simulink model "ZN_P1P2P3"  (R2019b)
settings: Solver=VariableStepAuto  StartTime=0.0  StopTime=300  RelTol=1e-3
libraries: simulink x3
settings Model: Creator=dibakarrajbongshi  LastModifiedBy=HP

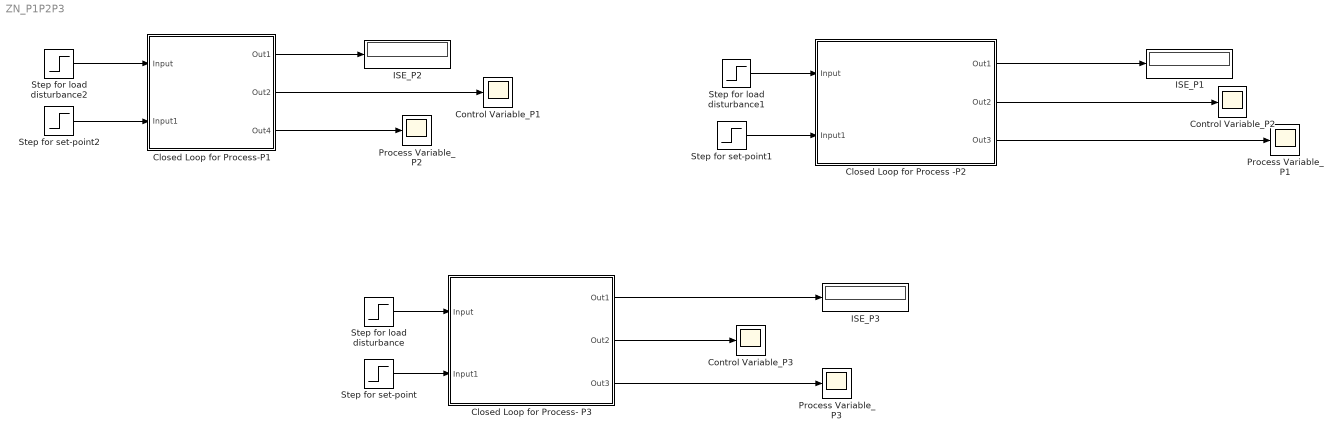
== system ZN_P1P2P3 ==
  Closed Loop for Process -P2 : Subsystem
  Closed Loop for Process- P3 : Subsystem
  Closed Loop for Process-P1 : Subsystem
  Control Variable_P1 : Scope
  Control Variable_P2 : Scope
  Control Variable_P3 : Scope
  ISE_P1 : Display
  ISE_P2 : Display
  ISE_P3 : Display
  Process Variable_P1 : Scope
  Process Variable_P2 : Scope
  Process Variable_P3 : Scope
  Step for load disturbance : Step  Time=0  After=0  SampleTime=0
  Step for load disturbance1 : Step  Time=0  After=0  SampleTime=0
  Step for load disturbance2 : Step  Time=0  After=0  SampleTime=0
  Step for set-point : Step  Time=0  SampleTime=0
  Step for set-point1 : Step  Time=0  SampleTime=0
  Step for set-point2 : Step  Time=0  SampleTime=0
  wires:
  Step for set-point2/1 -> Closed Loop for Process-P1/2(Input1)
  Closed Loop for Process-P1/3(Out4) -> Process Variable_P2/1
  Step for load disturbance2/1 -> Closed Loop for Process-P1/1(Input)
  Closed Loop for Process-P1/2(Out2) -> Control Variable_P1/1
  Closed Loop for Process-P1/1(Out1) -> ISE_P2/1
  Closed Loop for Process -P2/2(Out2) -> Control Variable_P2/1
  Step for load disturbance1/1 -> Closed Loop for Process -P2/1(Input)
  Closed Loop for Process -P2/3(Out3) -> Process Variable_P1/1
  Step for set-point1/1 -> Closed Loop for Process -P2/2(Input1)
  Closed Loop for Process -P2/1(Out1) -> ISE_P1/1
  Closed Loop for Process- P3/2(Out2) -> Control Variable_P3/1
  Closed Loop for Process- P3/3(Out3) -> Process Variable_P3/1
  Closed Loop for Process- P3/1(Out1) -> ISE_P3/1
  Step for load disturbance/1 -> Closed Loop for Process- P3/1(Input)
  Step for set-point/1 -> Closed Loop for Process- P3/2(Input1)

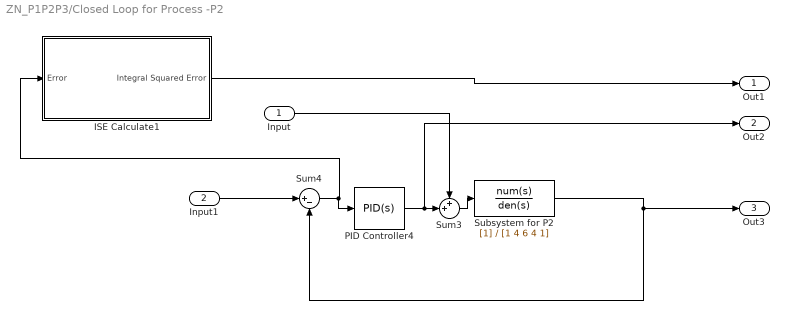
== system ZN_P1P2P3/Closed Loop for Process -P2 ==
  Input : Inport
  Input1 : Inport  Port=2
  ISE Calculate1 : Subsystem
  PID Controller4 : simulink/Continuous/PID Controller  Controller=PID  Form=Parallel  TimeDomain=Continuous-time  SampleTime=-1  IntegratorMethod=Forward Euler  FilterMethod=Forward Euler  ControllerParametersSource=internal  P=2.353  I=0.75  D=1.847  UseFilter=on  N=12.74  TunerSelectOption=Transfer Function Based (PID Tuner App)  InitialConditionSource=internal  InitialConditionForIntegrator=0  InitialConditionForFilter=0  DifferentiatorICPrevScaledInput=0  ExternalReset=none  TrackingMode=off  Kt=1  LimitOutput=off  UpperSaturationLimit=0.9  LowerSaturationLimit=0.1  LinearizeAsGain=on  AntiWindupMode=none  Kb=1  POutMin=[]  POutMax=[]  IOutMin=[]  IOutMax=[]  DOutMin=[]  DOutMax=[]  NOutMin=[]  NOutMax=[]  SumOutMin=[]  SumOutMax=[]  SaturationOutMin=[]  SaturationOutMax=[]  PParamMin=[]  PParamMax=[]  IParamMin=[]  IParamMax=[]  DParamMin=[]  DParamMax=[]  NParamMin=[]  NParamMax=[]  KbParamMin=[]  KbParamMax=[]  KtParamMin=[]  KtParamMax=[]  KbOutMin=[]  KbOutMax=[]  KtOutMin=[]  KtOutMax=[]  IntegratorOutMin=[]  IntegratorOutMax=[]  FilterOutMin=[]  FilterOutMax=[]  SumI1OutMin=[]  SumI1OutMax=[]  SumI2OutMin=[]  SumI2OutMax=[]  SumI3OutMin=[]  SumI3OutMax=[]  SumI4OutMin=[]  SumI4OutMax=[]  SumDOutMin=[]  SumDOutMax=[]  DifferentiatorOutMin=[]  DifferentiatorOutMax=[]  FilterDiffOutCoefMin=[]  FilterDiffOutCoefMax=[]  ReciprocalOutMin=[]  ReciprocalOutMax=[]  SumDenOutMin=[]  SumDenOutMax=[]  SumNumOutMin=[]  SumNumOutMax=[]  DivideOutMin=[]  DivideOutMax=[]  IntegratorContinuousStateAttributes=''  IntegratorStateMustResolveToSignalObject=off  IntegratorRTWStateStorageClass=Auto  FilterContinuousStateAttributes=''  FilterStateMustResolveToSignalObject=off  FilterRTWStateStorageClass=Auto  ParallelPVariant=InternalParameters  IdealPVariant=Disabled  IVariant=InternalParameters  DVariant=InternalParameters  IntegratorVariant=Continuous  SatVariant=Disabled  AWVariant=Passthrough  PCopyVariant=Disabled  TRVariant=Disabled  FdbkBlocksVariant=Forward  IdealPFdbkVariant=Disabled  SatFdbkVariant=Disabled  DerivativeFilterVariant=ContFilter  NVariant=InternalParameters  NCopyVariant=Disabled  FilterICVariant=InternalICsFilter  IntegratorICVariant=InternalICs  ExternalResetVariant=Disabled  TRSumVariant=Passthrough  SumFdbkVariant=Disabled  SumVariant=Sum_PID
  Subsystem for P2 : TransferFcn  Denominator=[1 4 6 4 1]
  Sum3 : Sum  Inputs=++|
  Sum4 : Sum  Inputs=|+-
  Out1 : Outport
  Out2 : Outport  Port=2
  Out3 : Outport  Port=3
  wires:
  PID Controller4/1 -> Out2/1, Sum3/2
  Input/1 -> Sum3/1
  Subsystem for P2/1 -> Out3/1, Sum4/2
  Sum4/1 -> PID Controller4/1, ISE Calculate1/1(Error)
  ISE Calculate1/1(Integral Squared Error) -> Out1/1
  Input1/1 -> Sum4/1
  Sum3/1 -> Subsystem for P2/1

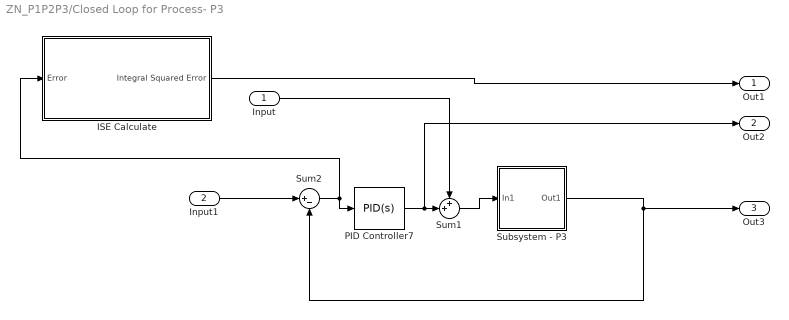
== system ZN_P1P2P3/Closed Loop for Process- P3 ==
  Input : Inport
  Input1 : Inport  Port=2
  ISE Calculate : Subsystem
  PID Controller7 : simulink/Continuous/PID Controller  Controller=PID  Form=Parallel  TimeDomain=Continuous-time  SampleTime=-1  IntegratorMethod=Forward Euler  FilterMethod=Forward Euler  ControllerParametersSource=internal  P=0.75  I=0.0382  D=3.6825  UseFilter=on  N=2.03666  TunerSelectOption=Transfer Function Based (PID Tuner App)  InitialConditionSource=internal  InitialConditionForIntegrator=0  InitialConditionForFilter=0  DifferentiatorICPrevScaledInput=0  ExternalReset=none  TrackingMode=off  Kt=1  LimitOutput=off  UpperSaturationLimit=0.9  LowerSaturationLimit=0.1  LinearizeAsGain=on  AntiWindupMode=none  Kb=1  POutMin=[]  POutMax=[]  IOutMin=[]  IOutMax=[]  DOutMin=[]  DOutMax=[]  NOutMin=[]  NOutMax=[]  SumOutMin=[]  SumOutMax=[]  SaturationOutMin=[]  SaturationOutMax=[]  PParamMin=[]  PParamMax=[]  IParamMin=[]  IParamMax=[]  DParamMin=[]  DParamMax=[]  NParamMin=[]  NParamMax=[]  KbParamMin=[]  KbParamMax=[]  KtParamMin=[]  KtParamMax=[]  KbOutMin=[]  KbOutMax=[]  KtOutMin=[]  KtOutMax=[]  IntegratorOutMin=[]  IntegratorOutMax=[]  FilterOutMin=[]  FilterOutMax=[]  SumI1OutMin=[]  SumI1OutMax=[]  SumI2OutMin=[]  SumI2OutMax=[]  SumI3OutMin=[]  SumI3OutMax=[]  SumI4OutMin=[]  SumI4OutMax=[]  SumDOutMin=[]  SumDOutMax=[]  DifferentiatorOutMin=[]  DifferentiatorOutMax=[]  FilterDiffOutCoefMin=[]  FilterDiffOutCoefMax=[]  ReciprocalOutMin=[]  ReciprocalOutMax=[]  SumDenOutMin=[]  SumDenOutMax=[]  SumNumOutMin=[]  SumNumOutMax=[]  DivideOutMin=[]  DivideOutMax=[]  IntegratorContinuousStateAttributes=''  IntegratorStateMustResolveToSignalObject=off  IntegratorRTWStateStorageClass=Auto  FilterContinuousStateAttributes=''  FilterStateMustResolveToSignalObject=off  FilterRTWStateStorageClass=Auto  ParallelPVariant=InternalParameters  IdealPVariant=Disabled  IVariant=InternalParameters  DVariant=InternalParameters  IntegratorVariant=Continuous  SatVariant=Disabled  AWVariant=Passthrough  PCopyVariant=Disabled  TRVariant=Disabled  FdbkBlocksVariant=Forward  IdealPFdbkVariant=Disabled  SatFdbkVariant=Disabled  DerivativeFilterVariant=ContFilter  NVariant=InternalParameters  NCopyVariant=Disabled  FilterICVariant=InternalICsFilter  IntegratorICVariant=InternalICs  ExternalResetVariant=Disabled  TRSumVariant=Passthrough  SumFdbkVariant=Disabled  SumVariant=Sum_PID
  Subsystem - P3 : Subsystem
  Sum1 : Sum  Inputs=++|
  Sum2 : Sum  Inputs=|+-
  Out1 : Outport
  Out2 : Outport  Port=2
  Out3 : Outport  Port=3
  wires:
  PID Controller7/1 -> Out2/1, Sum1/2
  Subsystem - P3/1(Out1) -> Out3/1, Sum2/2
  Sum2/1 -> PID Controller7/1, ISE Calculate/1(Error)
  ISE Calculate/1(Integral Squared Error) -> Out1/1
  Input1/1 -> Sum2/1
  Sum1/1 -> Subsystem - P3/1(In1)
  Input/1 -> Sum1/1

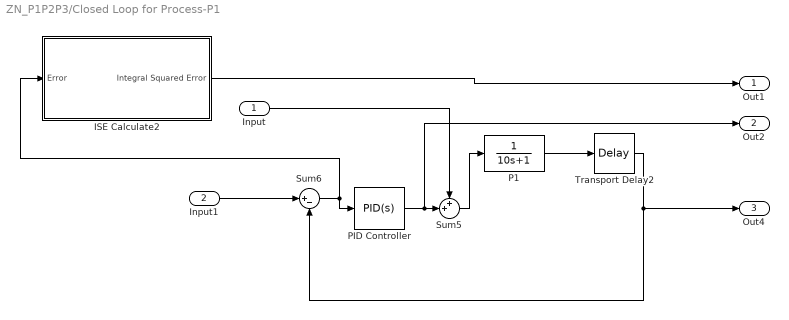
== system ZN_P1P2P3/Closed Loop for Process-P1 ==
  Input : Inport
  Input1 : Inport  Port=2
  ISE Calculate2 : Subsystem
  P1 : TransferFcn  Denominator=[10 1]
  PID Controller : simulink/Continuous/PID Controller  Controller=PID  Form=Parallel  TimeDomain=Continuous-time  SampleTime=-1  IntegratorMethod=Forward Euler  FilterMethod=Forward Euler  ControllerParametersSource=internal  P=2.676  I=0.449  D=3.99  UseFilter=on  N=6.711  TunerSelectOption=Transfer Function Based (PID Tuner App)  InitialConditionSource=internal  InitialConditionForIntegrator=0  InitialConditionForFilter=0  DifferentiatorICPrevScaledInput=0  ExternalReset=none  TrackingMode=off  Kt=1  LimitOutput=off  UpperSaturationLimit=0.9  LowerSaturationLimit=0.1  LinearizeAsGain=on  AntiWindupMode=none  Kb=1  POutMin=[]  POutMax=[]  IOutMin=[]  IOutMax=[]  DOutMin=[]  DOutMax=[]  NOutMin=[]  NOutMax=[]  SumOutMin=[]  SumOutMax=[]  SaturationOutMin=[]  SaturationOutMax=[]  PParamMin=[]  PParamMax=[]  IParamMin=[]  IParamMax=[]  DParamMin=[]  DParamMax=[]  NParamMin=[]  NParamMax=[]  KbParamMin=[]  KbParamMax=[]  KtParamMin=[]  KtParamMax=[]  KbOutMin=[]  KbOutMax=[]  KtOutMin=[]  KtOutMax=[]  IntegratorOutMin=[]  IntegratorOutMax=[]  FilterOutMin=[]  FilterOutMax=[]  SumI1OutMin=[]  SumI1OutMax=[]  SumI2OutMin=[]  SumI2OutMax=[]  SumI3OutMin=[]  SumI3OutMax=[]  SumI4OutMin=[]  SumI4OutMax=[]  SumDOutMin=[]  SumDOutMax=[]  DifferentiatorOutMin=[]  DifferentiatorOutMax=[]  FilterDiffOutCoefMin=[]  FilterDiffOutCoefMax=[]  ReciprocalOutMin=[]  ReciprocalOutMax=[]  SumDenOutMin=[]  SumDenOutMax=[]  SumNumOutMin=[]  SumNumOutMax=[]  DivideOutMin=[]  DivideOutMax=[]  IntegratorContinuousStateAttributes=''  IntegratorStateMustResolveToSignalObject=off  IntegratorRTWStateStorageClass=Auto  FilterContinuousStateAttributes=''  FilterStateMustResolveToSignalObject=off  FilterRTWStateStorageClass=Auto  ParallelPVariant=InternalParameters  IdealPVariant=Disabled  IVariant=InternalParameters  DVariant=InternalParameters  IntegratorVariant=Continuous  SatVariant=Disabled  AWVariant=Passthrough  PCopyVariant=Disabled  TRVariant=Disabled  FdbkBlocksVariant=Forward  IdealPFdbkVariant=Disabled  SatFdbkVariant=Disabled  DerivativeFilterVariant=ContFilter  NVariant=InternalParameters  NCopyVariant=Disabled  FilterICVariant=InternalICsFilter  IntegratorICVariant=InternalICs  ExternalResetVariant=Disabled  TRSumVariant=Passthrough  SumFdbkVariant=Disabled  SumVariant=Sum_PID
  Sum5 : Sum  Inputs=++|
  Sum6 : Sum  Inputs=|+-
  Transport Delay2 : TransportDelay  DelayTime=4  PadeOrder=1
  Out1 : Outport
  Out2 : Outport  Port=2
  Out4 : Outport  Port=3
  wires:
  Sum6/1 -> PID Controller/1, ISE Calculate2/1(Error)
  P1/1 -> Transport Delay2/1
  Input1/1 -> Sum6/1
  ISE Calculate2/1(Integral Squared Error) -> Out1/1
  PID Controller/1 -> Out2/1, Sum5/2
  Sum5/1 -> P1/1
  Transport Delay2/1 -> Out4/1, Sum6/2
  Input/1 -> Sum5/1

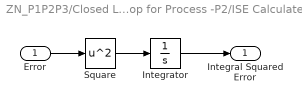
== system ZN_P1P2P3/Closed Loop for Process -P2/ISE Calculate1 ==
  Error : Inport
  Integrator : Integrator
  Square : Math  Operator=square  SignedPower=off  SaturateOnIntegerOverflow=on
  Integral Squared Error : Outport
  wires:
  Square/1 -> Integrator/1
  Error/1 -> Square/1
  Integrator/1 -> Integral Squared Error/1

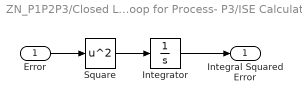
== system ZN_P1P2P3/Closed Loop for Process- P3/ISE Calculate ==
  Error : Inport
  Integrator : Integrator
  Square : Math  Operator=square  SignedPower=off  SaturateOnIntegerOverflow=on
  Integral Squared Error : Outport
  wires:
  Square/1 -> Integrator/1
  Error/1 -> Square/1
  Integrator/1 -> Integral Squared Error/1

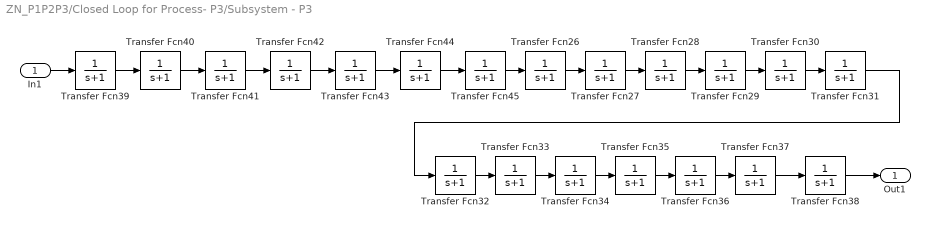
== system ZN_P1P2P3/Closed Loop for Process- P3/Subsystem - P3 ==
  In1 : Inport
  Transfer Fcn{26..45} (20 alike) : TransferFcn  Denominator=[1 1]
  Out1 : Outport
  wires:
  Transfer Fcn29/1 -> Transfer Fcn30/1
  Transfer Fcn43/1 -> Transfer Fcn44/1
  Transfer Fcn36/1 -> Transfer Fcn37/1
  Transfer Fcn33/1 -> Transfer Fcn34/1
  Transfer Fcn32/1 -> Transfer Fcn33/1
  Transfer Fcn35/1 -> Transfer Fcn36/1
  Transfer Fcn42/1 -> Transfer Fcn43/1
  Transfer Fcn37/1 -> Transfer Fcn38/1
  Transfer Fcn28/1 -> Transfer Fcn29/1
  Transfer Fcn27/1 -> Transfer Fcn28/1
  Transfer Fcn44/1 -> Transfer Fcn45/1
  Transfer Fcn41/1 -> Transfer Fcn42/1
  Transfer Fcn45/1 -> Transfer Fcn26/1
  Transfer Fcn26/1 -> Transfer Fcn27/1
  Transfer Fcn40/1 -> Transfer Fcn41/1
  Transfer Fcn30/1 -> Transfer Fcn31/1
  Transfer Fcn39/1 -> Transfer Fcn40/1
  Transfer Fcn38/1 -> Out1/1
  Transfer Fcn31/1 -> Transfer Fcn32/1
  Transfer Fcn34/1 -> Transfer Fcn35/1
  In1/1 -> Transfer Fcn39/1

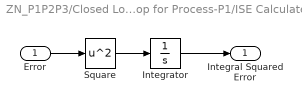
== system ZN_P1P2P3/Closed Loop for Process-P1/ISE Calculate2 ==
  Error : Inport
  Integrator : Integrator
  Square : Math  Operator=square  SignedPower=off  SaturateOnIntegerOverflow=on
  Integral Squared Error : Outport
  wires:
  Square/1 -> Integrator/1
  Error/1 -> Square/1
  Integrator/1 -> Integral Squared Error/1
